simulink model "BLDC_Ctrl_MBD"  (R2020b)
settings: Solver=FixedStepDiscrete  StartTime=0.0  StopTime=10.0  FixedStep=0.0001  RelTol=1e-3
PreLoadFcn:
  | load('struct_BLDC_Crtl.mat');
InitFcn:
  | mbd_s32k_consistency_checks(bdroot(gcs));
undefined symbols (not defined in the file): External, LQFP, One, Shot, TRGMUX_PDB_TRIG
libraries: mbd_s32k1xx_ec_toolbox x34, mcbcontrolslib x4, mbd_msd_ec_toolbox x1
(part 1 of 2)
settings Model: Creator=k  LastModifiedBy=k
settings DataIOCC: ExternalInput=off  InitialState=off  SaveOutput=off  SignalLogging=off  SaveTime=off
settings OptimizationCC: DefaultParameterBehavior=Inlined  EnhancedBackFolding=on  PassReuseOutputArgsAs=Individual arguments  ZeroExternalMemoryAtStartup=off  ZeroInternalMemoryAtStartup=off  OptimizeBlockOrder=speed  DifferentSizesBufferReuse=on  OptimizationCustomize=off  EfficientTunableParamExpr=on
settings DebuggingCC: InheritedTsInSrcMsg=none  SingleTaskRateTransMsg=error  ParameterTunabilityLossMsg=error  UnconnectedInputMsg=error  UnconnectedOutputMsg=error  UnconnectedLineMsg=error  UnknownTsInhSupMsg=error
settings HardwareCC: ProdBitPerPointer=32  ProdBitPerSizeT=32  ProdBitPerPtrDiffT=32  ProdLargestAtomicInteger=Long  ProdLargestAtomicFloat=Double  ProdWordSize=32  ProdHWDeviceType=ARM Compatible->ARM Cortex
settings ModelReferenceCC: ModelReferenceNumInstancesAllowed=Single
settings SFSimCC: MATLABDynamicMemAlloc=off
settings RTWCC: Description=Model Based Design Toolbox S32K1xx Code Generation Target  SystemTargetFile=mbd_s32k.tlc  MakeCommand=mbd_s32k_make_rtw COPY_MDLREF_INCLUDES=0  TemplateMakefile=mbd_s32k.tmf  GenerateReport=on
settings CodeAppCC: ForceParamTrailComments=on  IgnoreCustomStorageClasses=off  OperatorAnnotations=on  SimulinkDataObjDesc=on  SFDataObjDesc=on  InsertBlockDesc=on
settings STFCustomTargetCC: TargetLangStandard=C99 (ISO)  MultiwordLength=256  ConcurrentExecutionCompliant=off  CombineOutputUpdateFcns=on  ERTCustomFileBanners=on  SupportContinuousTime=off  SupportNonInlinedSFcns=off  RemoveResetFunc=on  MATLABClassNameForMDSCustomization=Simulink.SoftwareTarget.ERTCustomization  CPPClassGenCompliant=off  GRTInterface=off  SystemTargetFile=mbd_s32k.tlc
settings ERTTargetCC: TargetLangStandard=C99 (ISO)  ParMdlRefBuildCompliant=off  CompOptLevelCompliant=off  ConcurrentExecutionCompliant=off  ModelStepFunctionPrototypeControlCompliant=off  CPPClassGenCompliant=off  UseToolchainInfoCompliant=off  InlinedParameterPlacement=NonHierarchical  ERTSrcFileBannerTemplate=mbd_ert_code_template.cgt  ERTHdrFileBannerTemplate=mbd_ert_code_template.cgt  ERTDataSrcFileTemplate=mbd_ert_code_template.cgt  ERTDataHdrFileTemplate=mbd_ert_code_template.cgt  ERTCustomFileTemplate=example_file_process.tlc

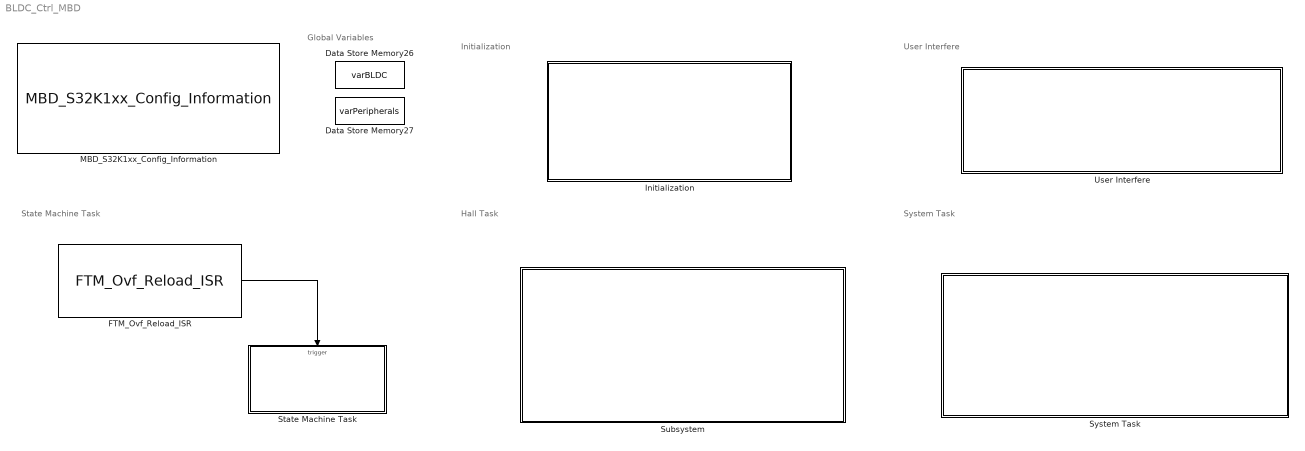
== system BLDC_Ctrl_MBD ==
  note: State Machine Task
  note: Global Variables
  note: Hall Task
  note: System Task
  note: Initialization
  note: User Interfere
  Data Store Memory26 : DataStoreMemory  DataStoreName=varBLDC  ReadBeforeWriteMsg=warning  WriteAfterWriteMsg=warning  WriteAfterReadMsg=warning  ShowAdditionalParam=off  OutDataTypeStr=Bus: structBLDC
  Data Store Memory27 : DataStoreMemory  DataStoreName=varPeripherals  ReadBeforeWriteMsg=warning  WriteAfterWriteMsg=warning  WriteAfterReadMsg=warning  ShowAdditionalParam=off  OutDataTypeStr=Bus: structPeripherals
  FTM_Ovf_Reload_ISR : mbd_s32k1xx_ec_toolbox/Motor Control Blocks/FTM Blocks/FTM_Ovf_Reload_ISR  Priority=10  ftmModule=3  mcuTargetUpdate=on
  Initialization : Subsystem
  MBD_S32K1xx_Config_Information : mbd_s32k1xx_ec_toolbox/MBD_S32K1xx_Config_Information  mbdt_ver=0  disp_str=|  config_params=[]  mcu_target_name=S32K144  mcu_target_package=100-LQFP  mcu_target_sram_size=64KB  mcu_system_clock_freq=80  mcu_xtal_freq=External 8  mcu_steptick_timer=LPIT Channel 0  mcu_steptick_prio=15  ds_import_enable=on  target_compiler=GCC  target_memory=FLASH  gcc_target_compile_opts=-mthumb -mfloat-abi=hard -mfpu=fpv4-sp-d16 -O1 -g -gstrict-dwarf  gcc_target_assemble_opts=-mthumb -mfloat-abi=hard -mfpu=fpv4-sp-d16 -g  gcc_target_link_opts=-mthumb -mfloat-abi=hard -mfpu=fpv4-sp-d16  gcc_target_default_lcf=on  gcc_target_user_lcf=S32K148_192_flash.ld  ghs_target_compile_opts=-cpu=cortexm4f -thumb -fpu=vfpv4_d16 -fsingle -Ogeneral -Wundef -Wimplicit-int -Wshadow -Wtrigraphs --no_commons --gnu_asm -gnu99 -gdwarf-2 -G  ghs_target_assemble_opts=-cpu=cortexm4f -fpu=vfpv4_d16  ghs_target_link_opts=-cpu=cortexm4f -thumb -fpu=vfpv4_d16  ghs_target_default_lcf=on  ghs_target_user_lcf=S32K148_192_flash.ld  iar_target_compile_opts=--cpu=Cortex-M4F --thumb --fpu=VFPv4_sp -Ol -e --debug --dlib_config normal  iar_target_assemble_opts=--cpu Cortex-M4F --thumb --fpu VFPv4_sp  iar_target_link_opts=--no_exceptions --vfe --inline  iar_target_default_lcf=on  iar_target_user_lcf=S32K148_192_flash.icf  pil_download_enable=off  rbl_download_enable=on  rbl_start_delay=5000  rbl_download_interface=OpenSDA  rbl_restart_request=off  rbl_com_port=Custom  rbl_com_port_custom=COM1  pil_download_rate=57600  pil_opensda_drive=Custom  pil_opensda_drive_custom=E  pil_uart_instance=1  pil_uart_rx=PTC6: [LPUART1_RX | Receive]  pil_uart_tx=PTC7: [LPUART1_TX | Transmit]  FTM_PWM_PcrCheckEnDis=on  FTM_Input_Edge_Inputs_PcrCheckEnDis=on  FTM_Dual_Edge_Inputs_PcrCheckEnDis=on  FTM_Quadrature_Inputs_PcrCheckEnDis=on  FTM_Hall_Sensor_Inputs_PcrCheckEnDis=on  LPTMR_PcrCheckEnDis=on  PIT_PcrCheckEnDis=on  RTC_PcrCheckEnDis=on  FlexCAN_PcrCheckEnDis=on  LIN_PcrCheckEnDis=on  FlexIO_PcrCheckEnDis=on  LPI2C_PcrCheckEnDis=on  LPSPI_PcrCheckEnDis=on  LPUART_PcrCheckEnDis=on  CMP_PcrCheckEnDis=on  GPIO_OutputPcrCheckEnDis=on  GPIO_InputPcrCheckEnDis=on  SBC_PcrCheckEnDis=on  BMS_PcrCheckEnDis=on  AMMCLIB_PcrCheckEnDis=on  FM_PcrCheckEnDis=on  Profile_PcrCheckEnDis=on  ConfigParams_PcrCheckEnDis=on  ModelRef_PcrCheckEnDis=on  PDB0_PcrCheckEnDis=on  CSEc_PcrCheckEnDis=on  eDMA_PcrCheckEnDis=on  FLASH_PcrCheckEnDis=on  ADC_PcrCheckEnDis=on  WDOG_PcrCheckEnDis=on
      | Target : S32K144-64KB_SRAM
      | Package : 100-pin
      | System clock : 80 MHz
      | XTAL clock : External 8 MHz
      | Compiler : IAR
      | Target Type : FLASH
      | Download Code after build : off
      | Step Tick Interrupt Priority : 15
  State Machine Task : Subsystem
  Subsystem : Subsystem
  System Task : Subsystem
  User Interfere : Subsystem
  wires:
  FTM_Ovf_Reload_ISR/1 -> State Machine Task/Trigger

== system BLDC_Ctrl_MBD/Initialization ==
  note: FreeMASTER
  note: ADC
  note: Configuration
  ADC_Config : mbd_s32k1xx_ec_toolbox/Motor Control Blocks/ADC Blocks/ADC_Config  instance=0  mode=12-bit conversion  smplts=20  adiclk=alternate clock 1  adiv=input clock  show_adv_opts=on  pretrgsel=PDB pre-trigger  swpretrg=Disabled  adtrg=hardware  trgsel=PDB output  refsel=Vrefh and Vrefl  supply_monitoring=off  acfe=off  acfgt=off  acren=off  cv1=0  cv2=0  adco=off  avge=off  avgs=4 samples
  ADC_Config1 : mbd_s32k1xx_ec_toolbox/Motor Control Blocks/ADC Blocks/ADC_Config  instance=1  mode=12-bit conversion  smplts=20  adiclk=alternate clock 1  adiv=input clock  show_adv_opts=on  pretrgsel=PDB pre-trigger  swpretrg=Disabled  adtrg=hardware  trgsel=PDB output  refsel=Vrefh and Vrefl  supply_monitoring=off  acfe=off  acfgt=off  acren=off  cv1=0  cv2=0  adco=off  avge=off  avgs=4 samples
  ADC_Interleave : mbd_s32k1xx_ec_toolbox/Motor Control Blocks/ADC Blocks/ADC_Interleave  adcInterleavePins=PTB1 to ADC0_SE5 and ADC1_SE15  adcInterleaveInit=on
  FreeMaster_Config : mbd_s32k1xx_ec_toolbox/Utility Blocks/FreeMaster_Config  interface=LPUART1  baudrate=115200  rxd=PTC6: [LPUART1_RX | Receive]  txd=PTC7: [LPUART1_TX | Transmit]  mode=Poll-driven  isr_prio=15  show_adv_opts=on  use_scope=on  max_scope_vars=8  use_recorder=on  max_rec_vars=8  rec_buff_size=8192  rec_timebase=50 milliseconds  comm_buffer_size_auto=on  comm_buffer_size=255  comm_rqueue_size_default=on  comm_rqueue_size=32
  "LPSPI_Config " : mbd_s32k1xx_ec_toolbox/Communication Blocks/SPI Blocks/LPSPI_Config   InstanceNumber=0  Role=Master  BaudRate=1000000  ShowAdvanced=on  sin=PTB3: [LPSPI0_SIN | LPSPI Serial Data Input]  sout=PTB4: [LPSPI0_SOUT | LPSPI Serial Data Output]  sck=PTB2: [LPSPI0_SCK | LPSPI Serial Clock I/O]  pcs0=None  pcs1=PTB5: [LPSPI0_PCS1 | Peripheral Chip Select 1]  pcs2=None  pcs3=None  CPHA=1  CPOL=0  BitOrder=MSB first  TransferSize=8  WhichPCS=0  PCSPol=ActiveLow  ContinuousTransfer=off
  PDB_Config : mbd_s32k1xx_ec_toolbox/Motor Control Blocks/PDB Blocks/PDB_Config  pdbModule=0  regScCont=One-Shot  regScTrgsel=External (TRGMUX_PDB_TRIG)  trgMuxSel=FTM3 Initialize Trigger  trgMuxSelPin=PTB5: [TRGMUX_IN0 | Trigger Mux Input]  regModModulus=3900  regScPrescaler=1  regScMult=1  regPoenPoen0=off  regPo0DlyDly1=0  regPo0DlyDly2=0  enable_pdb_init=on  show_adv_opts=on  regCh0C1En0=on  regCh0C1En1=on  regCh0C1En2=off  regCh0C1En3=off  regCh0C1En4=off  regCh0C1En5=off  regCh0C1En6=off  regCh0C1En7=off  regCh0C1Bb0=off  regCh0C1Bb1=off  regCh0C1Bb2=off  regCh0C1Bb3=off  regCh0C1Bb4=off  regCh0C1Bb5=off  regCh0C1Bb6=off  regCh0C1Bb7=off  regCh0C1Tos0=Pre-trigger is in delay mode  regCh0C1Tos1=Pre-trigger is in delay mode  regCh0C1Tos2=Pre-trigger is in delay mode  regCh0C1Tos3=Pre-trigger is in delay mode  regCh0C1Tos4=Pre-trigger is in delay mode  regCh0C1Tos5=Pre-trigger is in delay mode  regCh0C1Tos6=Pre-trigger is in delay mode  regCh0C1Tos7=Pre-trigger is in delay mode  regCh0DlyDly0=1500  regCh0DlyDly1=2000  regCh0DlyDly2=1000  regCh0DlyDly3=1500  regCh0DlyDly4=0  regCh0DlyDly5=0  regCh0DlyDly6=0  regCh0DlyDly7=0  regCh1C1En0=off  regCh1C1En1=off  regCh1C1En2=off  regCh1C1En3=off  regCh1C1En4=off  regCh1C1En5=off  regCh1C1En6=off  regCh1C1En7=off  regCh1C1Bb0=off  regCh1C1Bb1=off  regCh1C1Bb2=off  regCh1C1Bb3=off  regCh1C1Bb4=off  regCh1C1Bb5=off  regCh1C1Bb6=off  regCh1C1Bb7=off  regCh1C1Tos0=Pre-trigger is in delay mode  regCh1C1Tos1=Pre-trigger is in delay mode  regCh1C1Tos2=Pre-trigger is in delay mode  regCh1C1Tos3=Pre-trigger is in delay mode  regCh1C1Tos4=Pre-trigger is in delay mode  regCh1C1Tos5=Pre-trigger is in delay mode  regCh1C1Tos6=Pre-trigger is in delay mode  regCh1C1Tos7=Pre-trigger is in delay mode  regCh1DlyDly0=0  regCh1DlyDly1=0  regCh1DlyDly2=0  regCh1DlyDly3=0  regCh1DlyDly4=0  regCh1DlyDly5=0  regCh1DlyDly6=0  regCh1DlyDly7=0
  PDB_Config1 : mbd_s32k1xx_ec_toolbox/Motor Control Blocks/PDB Blocks/PDB_Config  pdbModule=1  regScCont=One-Shot  regScTrgsel=External (TRGMUX_PDB_TRIG)  trgMuxSel=FTM3 Initialize Trigger  trgMuxSelPin=PTB5: [TRGMUX_IN0 | Trigger Mux Input]  regModModulus=3900  regScPrescaler=1  regScMult=1  regPoenPoen0=off  regPo0DlyDly1=0  regPo0DlyDly2=0  enable_pdb_init=on  show_adv_opts=on  regCh0C1En0=on  regCh0C1En1=on  regCh0C1En2=on  regCh0C1En3=off  regCh0C1En4=off  regCh0C1En5=off  regCh0C1En6=off  regCh0C1En7=off  regCh0C1Bb0=off  regCh0C1Bb1=off  regCh0C1Bb2=off  regCh0C1Bb3=off  regCh0C1Bb4=off  regCh0C1Bb5=off  regCh0C1Bb6=off  regCh0C1Bb7=off  regCh0C1Tos0=Pre-trigger is in delay mode  regCh0C1Tos1=Pre-trigger is in delay mode  regCh0C1Tos2=Pre-trigger is in delay mode  regCh0C1Tos3=Pre-trigger is in delay mode  regCh0C1Tos4=Pre-trigger is in delay mode  regCh0C1Tos5=Pre-trigger is in delay mode  regCh0C1Tos6=Pre-trigger is in delay mode  regCh0C1Tos7=Pre-trigger is in delay mode  regCh0DlyDly0=1000  regCh0DlyDly1=1500  regCh0DlyDly2=2000  regCh0DlyDly3=0  regCh0DlyDly4=0  regCh0DlyDly5=0  regCh0DlyDly6=0  regCh0DlyDly7=0  regCh1C1En0=off  regCh1C1En1=off  regCh1C1En2=off  regCh1C1En3=off  regCh1C1En4=off  regCh1C1En5=off  regCh1C1En6=off  regCh1C1En7=off  regCh1C1Bb0=off  regCh1C1Bb1=off  regCh1C1Bb2=off  regCh1C1Bb3=off  regCh1C1Bb4=off  regCh1C1Bb5=off  regCh1C1Bb6=off  regCh1C1Bb7=off  regCh1C1Tos0=Pre-trigger is in delay mode  regCh1C1Tos1=Pre-trigger is in delay mode  regCh1C1Tos2=Pre-trigger is in delay mode  regCh1C1Tos3=Pre-trigger is in delay mode  regCh1C1Tos4=Pre-trigger is in delay mode  regCh1C1Tos5=Pre-trigger is in delay mode  regCh1C1Tos6=Pre-trigger is in delay mode  regCh1C1Tos7=Pre-trigger is in delay mode  regCh1DlyDly0=0  regCh1DlyDly1=0  regCh1DlyDly2=0  regCh1DlyDly3=0  regCh1DlyDly4=0  regCh1DlyDly5=0  regCh1DlyDly6=0  regCh1DlyDly7=0
  TPP_Config : mbd_msd_ec_toolbox/TPP/TPP_Config  Priority=1  tppInstance=0  desatMode=on  fullonMode=off  lockMode=off  overtempEvent=on  phaseEvent=off  desatEvent=off  framingEvent=on  vlsEvent=on  writeErrEvent=on  overcurrentEvent=on  resetEvent=on  mcuTppIntEn=off  prioInt=15  tppDeadtime=1500  initTppNow=on  tppSpiInst=Please add SPI block to workspace  tppPwmModule=Please add FTM block to workspace  tppPair0_1=on  tppPair2_3=on  tppPair4_5=on  tppPair6_7=off  tppFirstChHS=on  tppEn1Pin=PTA2: [PTA2 | Port A I/O]  tppEn2Pin=PTA2: [PTA2 | Port A I/O]  tppRstPin=PTA3: [PTA3 | Port A I/O]  tppCsPin=PTB5: [PTB5 | Port B I/O]  tppIntPin=PTE10: [PTE10 | Port E I/O]

== system BLDC_Ctrl_MBD/State Machine Task ==
  function : TriggerPort  TriggerType=function-call  VariantControl=Variant
  Chart : Stateflow chart  TreatAsAtomicUnit=on
      settings: PortSchema="{\"entries\":[{\"content\":{\"sides\":[{\"content\":{\"connectorIds\":[\"In1\",\"In2\"]},\"type\":\"ConnectorPlacement.EquallySpacedRectSide\",\"uuid\":\"6aab3670-dbd5-4778-9051-de706f320d6c\"},{\"content\":{\"connectorIds\":[\"Out7\",\"Out2\",\"Out3\",\"Out1\",\"Out4\",\"Out5\",\"Out6\",\"Out8\"],\"side\":\"RIGHT\"},\"type\":\"ConnectorPlacement.EquallySpacedRectSide\",\"uuid\":\"2f9f0170-7a01-4f36-b182-da63b20b6c86\"},{\"content\":{\"connectorIds\":[],\"side\":\"TOP\"},\"type\":\"ConnectorPlacement.EquallySpacedRectSide\",\"uuid\":\"ed2088fa-8282-455e-b501-bc381afe58e4\"},{\"content\":{\"connectorIds\":[],\"side\":\"HIDDEN\"},\"type\":\"ConnectorPlacement.EquallySpacedRectSide\",\"uuid\":\"d652818b-6052-4db5-9e3c-1b8d8b3f5bf8\"}]},\"type\":\"ConnectorPlacement.EquallySpacedConnector\",\"uuid\":\"e57e4f41-1290-4580-a9fc-0c62073a8c32\"}],\"packageUris\":[\"http://schema.mathworks.com/mf0/Connector/R2020b\"],\"version\":\"1.0\"}"
  Data Store Read1 : DataStoreRead  DataStoreName=varBLDC  DataStoreElements=varBLDC.varMotorCtrl.FaultSetClear
  Data Store Read3 : DataStoreRead  DataStoreName=varBLDC  DataStoreElements=varBLDC.varMotorCtrl.MotorOnOff
  FreeMaster_Recorder_Call : mbd_s32k1xx_ec_toolbox/Utility Blocks/FreeMaster_Recorder_Call
  Read ADC : Subsystem
  State Functions : Subsystem  Priority=1
  Update FTM : Subsystem
  wires:
  Chart/7(ReadADCFunc()) -> Read ADC/Trigger
  Data Store Read1/1 -> Chart/2(FaultSetClear)
  Chart/8(UpdateFTMFunc()) -> Update FTM/Trigger
  Chart/6(FaultFunc()) -> State Functions/6(FaultFuncCall)
  Chart/3(ReadyFunc()) -> State Functions/2(ReadyFuncCall)
  Chart/5(NormalRunFunc()) -> State Functions/5(NomalRunFuncCall)
  Chart/1(MeasFunc()) -> State Functions/3(MeasFuncCall)
  Chart/2(InitFunc()) -> State Functions/1(InitFuncCall)
  Chart/4(CalFunc()) -> State Functions/4(CalFuncCall)
  Data Store Read3/1 -> Chart/1(MotorOnOff)

== system BLDC_Ctrl_MBD/Subsystem ==
  Digital_Input_ISR : mbd_s32k1xx_ec_toolbox/GPIO Blocks/Digital_Input_ISR  gpio_pin=PTA1: [PTA1 | Port A I/O]  irqc=on either-edge  prio=5
  Digital_Input_ISR1 : mbd_s32k1xx_ec_toolbox/GPIO Blocks/Digital_Input_ISR  gpio_pin=PTA15: [PTA15 | Port A I/O]  irqc=on either-edge  prio=5
  Digital_Input_ISR2 : mbd_s32k1xx_ec_toolbox/GPIO Blocks/Digital_Input_ISR  gpio_pin=PTA16: [PTA16 | Port A I/O]  irqc=on either-edge  prio=5
  Hall A : Subsystem  TreatAsAtomicUnit=on
  Hall B : Subsystem  TreatAsAtomicUnit=on
  Hall C : Subsystem  TreatAsAtomicUnit=on
  wires:
  Digital_Input_ISR/1 -> Hall C/Trigger
  Digital_Input_ISR1/1 -> Hall A/Trigger
  Digital_Input_ISR2/1 -> Hall B/Trigger

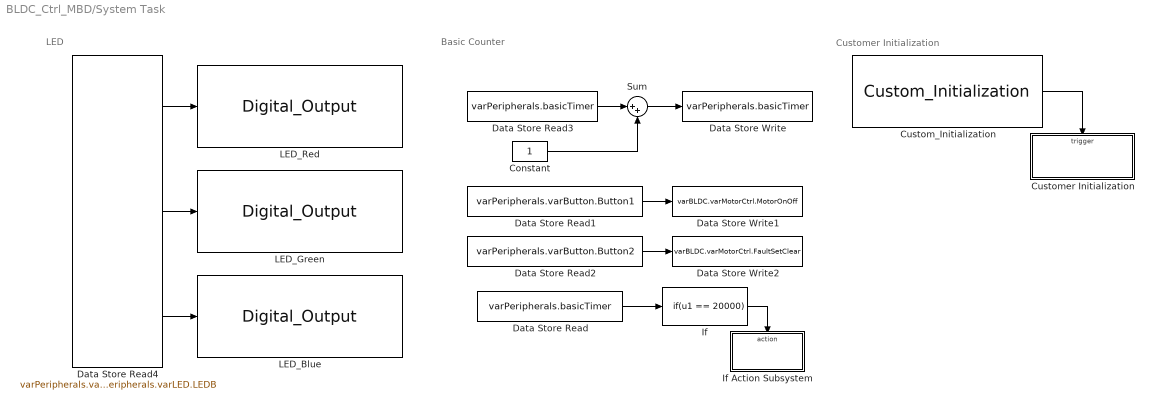
== system BLDC_Ctrl_MBD/System Task ==
  note: LED
  note: Basic Counter
  note: Customer Initialization
  Constant : Constant  OutDataTypeStr=uint32
  Custom_Initialization : mbd_s32k1xx_ec_toolbox/Utility Blocks/Custom_Initialization
  Customer Initialization : Subsystem  TreatAsAtomicUnit=on
  Data Store Read : DataStoreRead  DataStoreName=varPeripherals  DataStoreElements=varPeripherals.basicTimer
  Data Store Read1 : DataStoreRead  DataStoreName=varPeripherals  DataStoreElements=varPeripherals.varButton.Button1
  Data Store Read2 : DataStoreRead  DataStoreName=varPeripherals  DataStoreElements=varPeripherals.varButton.Button2
  Data Store Read3 : DataStoreRead  DataStoreName=varPeripherals  DataStoreElements=varPeripherals.basicTimer
  Data Store Read4 : DataStoreRead  DataStoreName=varPeripherals  DataStoreElements=varPeripherals.varLED.LEDR#varPeripherals.varLED.LEDG#varPeripherals.varLED.LEDB
  Data Store Write : DataStoreWrite  DataStoreName=varPeripherals  DataStoreElements=varPeripherals.basicTimer
  Data Store Write1 : DataStoreWrite  DataStoreName=varBLDC  DataStoreElements=varBLDC.varMotorCtrl.MotorOnOff
  Data Store Write2 : DataStoreWrite  DataStoreName=varBLDC  DataStoreElements=varBLDC.varMotorCtrl.FaultSetClear
  If : If  IfExpression=u1 == 20000  ShowElse=off
  If Action Subsystem : Subsystem  TreatAsAtomicUnit=on
  LED_Blue : mbd_s32k1xx_ec_toolbox/GPIO Blocks/Digital_Output  gpio_pin=PTD0: [PTD0 | Port D I/O]  init_val=High  drive_strength=Low
  LED_Green : mbd_s32k1xx_ec_toolbox/GPIO Blocks/Digital_Output  gpio_pin=PTD16: [PTD16 | Port D I/O]  init_val=High  drive_strength=Low
  LED_Red : mbd_s32k1xx_ec_toolbox/GPIO Blocks/Digital_Output  gpio_pin=PTD15: [PTD15 | Port D I/O]  init_val=High  drive_strength=Low
  Sum : Sum  Inputs=|++
  wires:
  Data Store Read4/1 -> LED_Red/1
  Data Store Read4/2 -> LED_Green/1
  Data Store Read4/3 -> LED_Blue/1
  Constant/1 -> Sum/2
  Sum/1 -> Data Store Write/1
  Custom_Initialization/1 -> Customer Initialization/Trigger
  Data Store Read1/1 -> Data Store Write1/1
  Data Store Read2/1 -> Data Store Write2/1
  Data Store Read/1 -> If/1
  If/1 -> If Action Subsystem/Action
  Data Store Read3/1 -> Sum/1

== system BLDC_Ctrl_MBD/User Interfere ==
  note: User Button
  note: User PIT Task
  Digital_Input_ISR : mbd_s32k1xx_ec_toolbox/GPIO Blocks/Digital_Input_ISR  gpio_pin=PTC12: [PTC12 | Port C I/O]  irqc=on rising-edge  prio=13
  Digital_Input_ISR1 : mbd_s32k1xx_ec_toolbox/GPIO Blocks/Digital_Input_ISR  gpio_pin=PTC13: [PTC13 | Port C I/O]  irqc=on rising-edge  prio=13
  Function-Call Subsystem1 : Subsystem  TreatAsAtomicUnit=on
  Function-Call Subsystem2 : Subsystem  TreatAsAtomicUnit=on
  Periodic_Interrupt_Timer : mbd_s32k1xx_ec_toolbox/Utility Blocks/Periodic_Interrupt_Timer  channel=1  period=200  prio=14  startCounter=on
  User PIT Task : Subsystem  TreatAsAtomicUnit=on
  wires:
  Digital_Input_ISR/1 -> Function-Call Subsystem2/Trigger
  Digital_Input_ISR1/1 -> Function-Call Subsystem1/Trigger
  Periodic_Interrupt_Timer/1 -> User PIT Task/Trigger

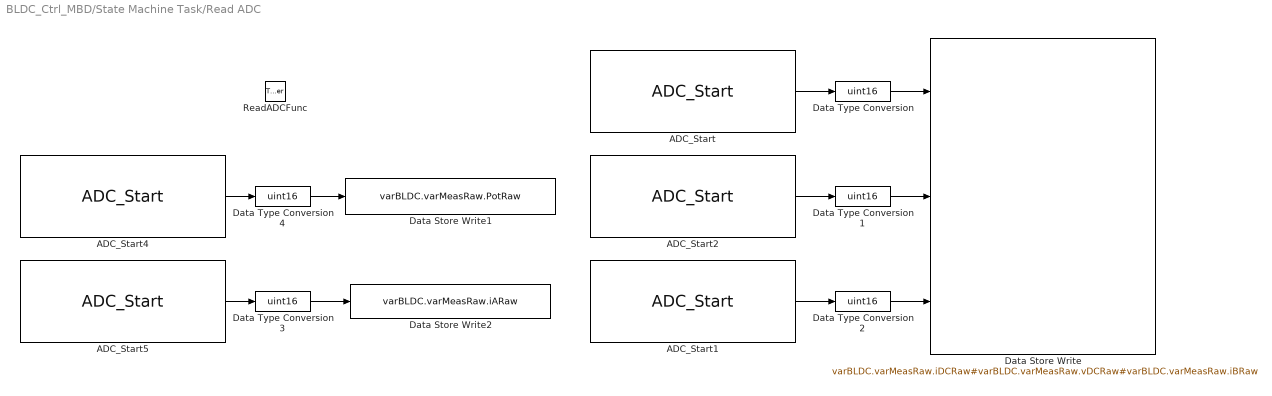
== system BLDC_Ctrl_MBD/State Machine Task/Read ADC ==
  ReadADCFunc : TriggerPort  TriggerType=function-call  VariantControl=Variant
  ADC_Start : mbd_s32k1xx_ec_toolbox/Motor Control Blocks/ADC Blocks/ADC_Start  instance=1  adc_r=A  adc_chan=PTD4: [ADC1_SE6 | ADC Single Ended Input]  aien=off  mcuTargetUpdate=on
  ADC_Start1 : mbd_s32k1xx_ec_toolbox/Motor Control Blocks/ADC Blocks/ADC_Start  instance=1  adc_r=C  adc_chan=PTB1: [ADC1_SE15 | ADC Single Ended Input]  aien=off  mcuTargetUpdate=on
  ADC_Start2 : mbd_s32k1xx_ec_toolbox/Motor Control Blocks/ADC Blocks/ADC_Start  instance=1  adc_r=B  adc_chan=PTB12: [ADC1_SE7 | ADC Single Ended Input]  aien=off  mcuTargetUpdate=on
  ADC_Start4 : mbd_s32k1xx_ec_toolbox/Motor Control Blocks/ADC Blocks/ADC_Start  instance=0  adc_r=A  adc_chan=PTC14: [ADC0_SE12 | ADC Single Ended Input]  aien=off  mcuTargetUpdate=on
  ADC_Start5 : mbd_s32k1xx_ec_toolbox/Motor Control Blocks/ADC Blocks/ADC_Start  instance=0  adc_r=B  adc_chan=PTB0: [ADC0_SE4 | ADC Single Ended Input]  aien=off  mcuTargetUpdate=on
  Data Store Write : DataStoreWrite  DataStoreName=varBLDC  DataStoreElements=varBLDC.varMeasRaw.iDCRaw#varBLDC.varMeasRaw.vDCRaw#varBLDC.varMeasRaw.iBRaw
  Data Store Write1 : DataStoreWrite  DataStoreName=varBLDC  DataStoreElements=varBLDC.varMeasRaw.PotRaw
  Data Store Write2 : DataStoreWrite  DataStoreName=varBLDC  DataStoreElements=varBLDC.varMeasRaw.iARaw
  Data Type Conversion{,1..4} (5 alike) : DataTypeConversion  OutDataTypeStr=uint16
  wires:
  ADC_Start5/1 -> Data Type Conversion3/1
  ADC_Start/1 -> Data Type Conversion/1
  ADC_Start1/1 -> Data Type Conversion2/1
  Data Type Conversion/1 -> Data Store Write/1
  ADC_Start4/1 -> Data Type Conversion4/1
  Data Type Conversion4/1 -> Data Store Write1/1
  ADC_Start2/1 -> Data Type Conversion1/1
  Data Type Conversion3/1 -> Data Store Write2/1
  Data Type Conversion2/1 -> Data Store Write/3
  Data Type Conversion1/1 -> Data Store Write/2

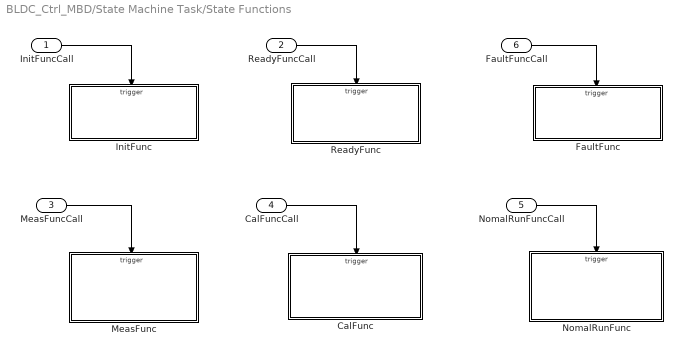
== system BLDC_Ctrl_MBD/State Machine Task/State Functions ==
  InitFuncCall : Inport
  ReadyFuncCall : Inport  Port=2
  MeasFuncCall : Inport  Port=3
  CalFuncCall : Inport  Port=4
  NomalRunFuncCall : Inport  Port=5
  FaultFuncCall : Inport  Port=6
  CalFunc : Subsystem  TreatAsAtomicUnit=on
  FaultFunc : Subsystem  TreatAsAtomicUnit=on
  InitFunc : Subsystem  TreatAsAtomicUnit=on
  MeasFunc : Subsystem  TreatAsAtomicUnit=on
  NomalRunFunc : Subsystem  TreatAsAtomicUnit=on
  ReadyFunc : Subsystem  TreatAsAtomicUnit=on
  wires:
  MeasFuncCall/1 -> MeasFunc/Trigger
  CalFuncCall/1 -> CalFunc/Trigger
  InitFuncCall/1 -> InitFunc/Trigger
  ReadyFuncCall/1 -> ReadyFunc/Trigger
  FaultFuncCall/1 -> FaultFunc/Trigger
  NomalRunFuncCall/1 -> NomalRunFunc/Trigger

== system BLDC_Ctrl_MBD/State Machine Task/Update FTM ==
  UpdateFTMFunc : TriggerPort  TriggerType=function-call  VariantControl=Variant
  Data Store Read2 : DataStoreRead  DataStoreName=varBLDC  DataStoreElements=varBLDC.varDuty.DutyA#varBLDC.varDuty.DutyB#varBLDC.varDuty.DutyC#varBLDC.varDuty.SWOCTRLcode#varBLDC.varDuty.OUTMASKcode
  FTM_PWM_Config : mbd_s32k1xx_ec_toolbox/Motor Control Blocks/FTM Blocks/FTM_PWM_Config  Priority=5  ftmModule=3  ftmMode=Center-Aligned PWM  ftmSourceClock=80 MHz  swcontrol_enable=on  chan0En=on  chan0Type=Complementary  chan2En=on  chan2Type=Complementary  chan4En=on  chan4Type=Complementary  chan6En=off  chan6Type=Independent  ftmPwmUnits=Hz  outFrequency=20000  ftmPeriod=4000  ftmPrescaler=Divide by 1  deadtimeUnits=Nanoseconds  deadtimeNs=1200  deadtimeTicks=24  deadtimePrescaler=Divide by 4  dutyCycleCh0=0  dutyCycleCh1=0  dutyCycleCh2=0  dutyCycleCh3=0  dutyCycleCh4=0  dutyCycleCh5=0  dutyCycleCh6=0.25  dutyCycleCh7=0.25  dutyCycleSim=off  startAfterInit=off  showAdvOpt=on  pinFtmCh0=PTB8: [FTM3_CH0 | FTM Channel]  pinFtmCh1=PTB9: [FTM3_CH1 | FTM Channel]  pinPolCh0=Active Low  pinPolCh1=Active Low  outputComplem0=Main duplicated  outputLevel0=High  outputLevel1=Low  pinFtmCh2=PTB10: [FTM3_CH2 | FTM Channel]  pinFtmCh3=PTB11: [FTM3_CH3 | FTM Channel]  pinPolCh2=Active Low  pinPolCh3=Active Low  outputComplem2=Main duplicated  outputLevel2=High  outputLevel3=Low  pinFtmCh4=PTC10: [FTM3_CH4 | FTM Channel]  pinFtmCh5=PTC11: [FTM3_CH5 | FTM Channel]  pinPolCh4=Active Low  pinPolCh5=Active Low  outputComplem4=Main duplicated  outputLevel4=High  outputLevel5=Low  pinFtmCh6=PTC12: [FTM3_CH6 | FTM Channel]  pinFtmCh7=None  pinPolCh6=Active Low  pinPolCh7=Active Low  outputComplem6=Main duplicated  outputLevel6=Low  outputLevel7=Low  initTrigger=off  chTrigger0=off  chTrigger1=off  chTrigger2=off  chTrigger3=off  chTrigger4=off  chTrigger5=off  chTrigger6=off  chTrigger7=off  mcuTargetUpdate=on  pwmSyncTrg=Software trigger  pwmSyncHwRouting=TRGMUX_FTM7  pwmSyncTrg0=off  pwmSyncTrg1=off  pwmSyncTrg2=off  pwmSyncAutoClear=off  pwmSyncMinLoad=on  pwmSyncMaxLoad=off  pwmSyncInvert=PWM Syncronization  pwmSyncOutControl=System Clock  pwmSyncOutMask=System Clock  pwmSyncCounterInitial=PWM Syncronization  pwmSyncPoints=Wait Loading Points  reloadEnable=on  reloadPriority=5  reloadHalfCycle=off  reloadHCR=0  reloadFrequency=0  chnMatch0=off  chnMatch1=off  chnMatch2=off  chnMatch3=off  chnMatch4=off  chnMatch5=off  chnMatch6=off  chnMatch7=off  pwmFaultProtection=off  pwmFaultInterrupt=off  pwmFaultClearing=Fault control disabled  pwmFaultPinState=Safe Value  pwmFaultFilterValue=0  pwmFaultPriority=15  fault_disen_0=off  fault_filter_0=off  fault_polarity_0=Active High  fault_disen_1=off  fault_filter_1=off  fault_polarity_1=Active high  fault_disen_2=off  fault_filter_2=off  fault_polarity_2=Active high  fault_disen_3=off  fault_filter_3=off  fault_polarity_3=Active high  fault_pin_0=None  fault_pin_1=None  fault_pin_2=None  fault_pin_3=None
  wires:
  Data Store Read2/1 -> FTM_PWM_Config/1
  Data Store Read2/3 -> FTM_PWM_Config/3
  Data Store Read2/2 -> FTM_PWM_Config/2
  Data Store Read2/4 -> FTM_PWM_Config/4
  Data Store Read2/5 -> FTM_PWM_Config/5

== system BLDC_Ctrl_MBD/Subsystem/Hall A ==
  ReadHallA : TriggerPort  TriggerType=function-call  VariantControl=Variant
  Data Store Read1 : DataStoreRead  DataStoreName=varBLDC  DataStoreElements=varBLDC.varHallCalc.HallEnd
  Data Store Read5 : DataStoreRead  DataStoreName=varPeripherals  DataStoreElements=varPeripherals.basicTimer
  Data Store Write1 : DataStoreWrite  DataStoreName=varBLDC  DataStoreElements=varBLDC.varHall.HallA
  Data Store Write2 : DataStoreWrite  DataStoreName=varBLDC  DataStoreElements=varBLDC.varHallCalc.HallEnd
  Data Store Write3 : DataStoreWrite  DataStoreName=varBLDC  DataStoreElements=varBLDC.varHallCalc.HallStart
  Digital_Input_HALL_A : mbd_s32k1xx_ec_toolbox/GPIO Blocks/Digital_Input  gpio_pin=PTA15: [PTA15 | Port A I/O]  pull_resistor=None  passive_filter=off
  wires:
  Digital_Input_HALL_A/1 -> Data Store Write1/1
  Data Store Read1/1 -> Data Store Write3/1
  Data Store Read5/1 -> Data Store Write2/1

== system BLDC_Ctrl_MBD/Subsystem/Hall B ==
  ReadHallA : TriggerPort  TriggerType=function-call  VariantControl=Variant
  Data Store Read1 : DataStoreRead  DataStoreName=varBLDC  DataStoreElements=varBLDC.varHallCalc.HallEnd
  Data Store Read5 : DataStoreRead  DataStoreName=varPeripherals  DataStoreElements=varPeripherals.basicTimer
  Data Store Write1 : DataStoreWrite  DataStoreName=varBLDC  DataStoreElements=varBLDC.varHall.HallB
  Data Store Write2 : DataStoreWrite  DataStoreName=varBLDC  DataStoreElements=varBLDC.varHallCalc.HallEnd
  Data Store Write3 : DataStoreWrite  DataStoreName=varBLDC  DataStoreElements=varBLDC.varHallCalc.HallStart
  Digital_Input_HALL_B : mbd_s32k1xx_ec_toolbox/GPIO Blocks/Digital_Input  gpio_pin=PTA16: [PTA16 | Port A I/O]  pull_resistor=None  passive_filter=off
  wires:
  Digital_Input_HALL_B/1 -> Data Store Write1/1
  Data Store Read5/1 -> Data Store Write2/1
  Data Store Read1/1 -> Data Store Write3/1

== system BLDC_Ctrl_MBD/Subsystem/Hall C ==
  ReadHallA : TriggerPort  TriggerType=function-call  VariantControl=Variant
  Data Store Read1 : DataStoreRead  DataStoreName=varBLDC  DataStoreElements=varBLDC.varHallCalc.HallEnd
  Data Store Read5 : DataStoreRead  DataStoreName=varPeripherals  DataStoreElements=varPeripherals.basicTimer
  Data Store Write1 : DataStoreWrite  DataStoreName=varBLDC  DataStoreElements=varBLDC.varHall.HallC
  Data Store Write2 : DataStoreWrite  DataStoreName=varBLDC  DataStoreElements=varBLDC.varHallCalc.HallEnd
  Data Store Write3 : DataStoreWrite  DataStoreName=varBLDC  DataStoreElements=varBLDC.varHallCalc.HallStart
  Digital_Input_HALL_C : mbd_s32k1xx_ec_toolbox/GPIO Blocks/Digital_Input  gpio_pin=PTA1: [PTA1 | Port A I/O]  pull_resistor=None  passive_filter=off
  wires:
  Digital_Input_HALL_C/1 -> Data Store Write1/1
  Data Store Read5/1 -> Data Store Write2/1
  Data Store Read1/1 -> Data Store Write3/1

== system BLDC_Ctrl_MBD/System Task/Customer Initialization ==
  CustInit : TriggerPort  TriggerType=function-call  VariantControl=Variant
  0_uint32 : Constant  Value=0  OutDataTypeStr=uint32
  1_boolean : Constant  OutDataTypeStr=boolean
  Data Store Write : DataStoreWrite  DataStoreName=varPeripherals  DataStoreElements=varPeripherals.varLED.LEDR#varPeripherals.varLED.LEDG#varPeripherals.varLED.LEDB#varPeripherals.basicTimer
  wires:
  1_boolean/1 -> Data Store Write/1, Data Store Write/2, Data Store Write/3
  0_uint32/1 -> Data Store Write/4

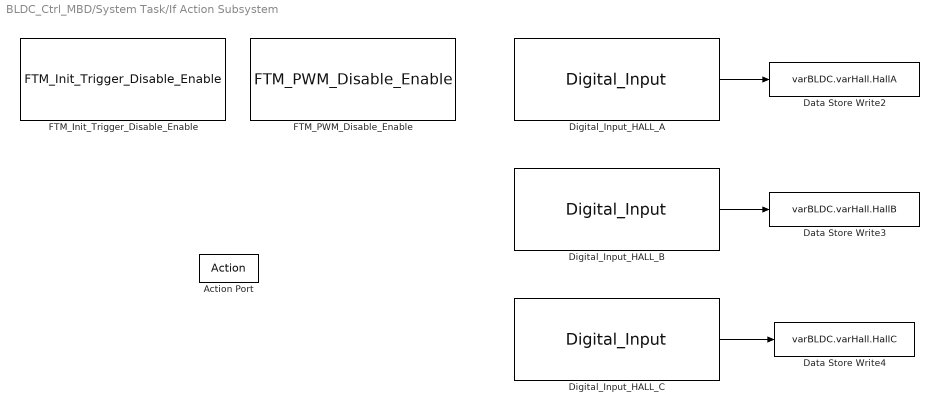
== system BLDC_Ctrl_MBD/System Task/If Action Subsystem ==
  Action Port : ActionPort  ActionPortLabel=if(u1 == 20000)
  Data Store Write2 : DataStoreWrite  DataStoreName=varBLDC  DataStoreElements=varBLDC.varHall.HallA
  Data Store Write3 : DataStoreWrite  DataStoreName=varBLDC  DataStoreElements=varBLDC.varHall.HallB
  Data Store Write4 : DataStoreWrite  DataStoreName=varBLDC  DataStoreElements=varBLDC.varHall.HallC
  Digital_Input_HALL_A : mbd_s32k1xx_ec_toolbox/GPIO Blocks/Digital_Input  gpio_pin=PTA15: [PTA15 | Port A I/O]  pull_resistor=None  passive_filter=off
  Digital_Input_HALL_B : mbd_s32k1xx_ec_toolbox/GPIO Blocks/Digital_Input  gpio_pin=PTA16: [PTA16 | Port A I/O]  pull_resistor=None  passive_filter=off
  Digital_Input_HALL_C : mbd_s32k1xx_ec_toolbox/GPIO Blocks/Digital_Input  gpio_pin=PTA1: [PTA1 | Port A I/O]  pull_resistor=None  passive_filter=off
  FTM_Init_Trigger_Disable_Enable : mbd_s32k1xx_ec_toolbox/Motor Control Blocks/FTM Blocks/FTM_Init_Trigger_Disable_Enable  ftmModule=3  action=Enable
  FTM_PWM_Disable_Enable : mbd_s32k1xx_ec_toolbox/Motor Control Blocks/FTM Blocks/FTM_PWM_Disable_Enable  ftmModule=3  action=Enable
  wires:
  Digital_Input_HALL_A/1 -> Data Store Write2/1
  Digital_Input_HALL_B/1 -> Data Store Write3/1
  Digital_Input_HALL_C/1 -> Data Store Write4/1

== system BLDC_Ctrl_MBD/User Interfere/Function-Call Subsystem1 ==
  function : TriggerPort  TriggerType=function-call  VariantControl=Variant
  Data Store Read : DataStoreRead  DataStoreName=varPeripherals  DataStoreElements=varPeripherals.varButton.Button2
  Data Store Write : DataStoreWrite  DataStoreName=varPeripherals  DataStoreElements=varPeripherals.varButton.Button2
  Logical Operator : Logic  Operator=NOT  AllPortsSameDT=off  OutDataTypeStr=boolean
  wires:
  Data Store Read/1 -> Logical Operator/1
  Logical Operator/1 -> Data Store Write/1

== system BLDC_Ctrl_MBD/User Interfere/Function-Call Subsystem2 ==
  function : TriggerPort  TriggerType=function-call  VariantControl=Variant
  Data Store Read : DataStoreRead  DataStoreName=varPeripherals  DataStoreElements=varPeripherals.varButton.Button1
  Data Store Write : DataStoreWrite  DataStoreName=varPeripherals  DataStoreElements=varPeripherals.varButton.Button1
  Logical Operator : Logic  Operator=NOT  AllPortsSameDT=off  OutDataTypeStr=boolean
  wires:
  Logical Operator/1 -> Data Store Write/1
  Data Store Read/1 -> Logical Operator/1

== system BLDC_Ctrl_MBD/User Interfere/User PIT Task ==
  UserPITFunc : TriggerPort  TriggerType=function-call  VariantControl=Variant
  Constant : Constant  Value=0.168  OutDataTypeStr=single
  Data Store Read : DataStoreRead  DataStoreName=varBLDC  DataStoreElements=varBLDC.varMeasRaw.PotRaw
  Data Store Write1 : DataStoreWrite  DataStoreName=varBLDC  DataStoreElements=varBLDC.varMotorCtrl.SpdReq
  Data Type Conversion : DataTypeConversion  OutDataTypeStr=single
  Product : Product
  Saturation : Saturate  UpperLimit=650  LowerLimit=0
  wires:
  Saturation/1 -> Data Store Write1/1
  Data Store Read/1 -> Data Type Conversion/1
  Data Type Conversion/1 -> Product/1
  Constant/1 -> Product/2
  Product/1 -> Saturation/1

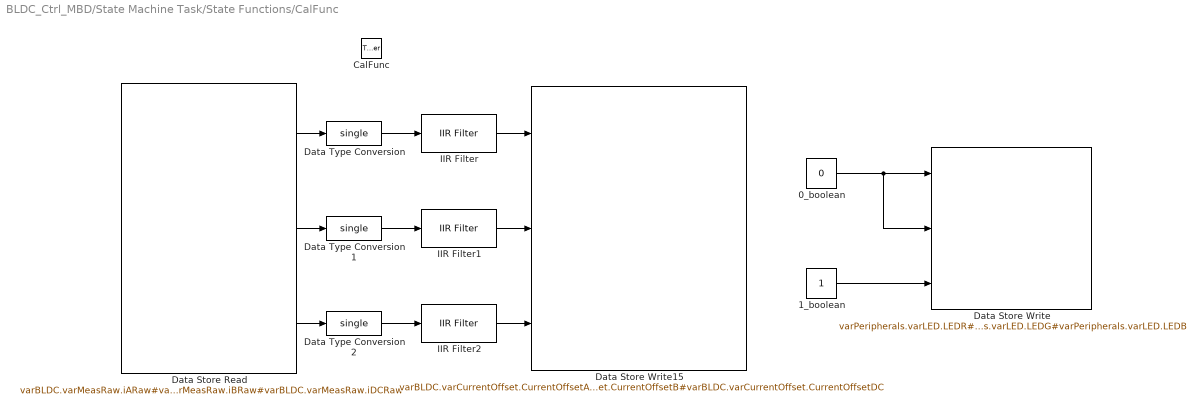
== system BLDC_Ctrl_MBD/State Machine Task/State Functions/CalFunc ==
  CalFunc : TriggerPort  TriggerType=function-call  VariantControl=Variant
  0_boolean : Constant  Value=0  OutDataTypeStr=boolean
  1_boolean : Constant  OutDataTypeStr=boolean
  Data Store Read : DataStoreRead  DataStoreName=varBLDC  DataStoreElements=varBLDC.varMeasRaw.iARaw#varBLDC.varMeasRaw.iBRaw#varBLDC.varMeasRaw.iDCRaw
  Data Store Write : DataStoreWrite  DataStoreName=varPeripherals  DataStoreElements=varPeripherals.varLED.LEDR#varPeripherals.varLED.LEDG#varPeripherals.varLED.LEDB
  Data Store Write15 : DataStoreWrite  DataStoreName=varBLDC  DataStoreElements=varBLDC.varCurrentOffset.CurrentOffsetA#varBLDC.varCurrentOffset.CurrentOffsetB#varBLDC.varCurrentOffset.CurrentOffsetDC
  Data Type Conversion : DataTypeConversion  OutDataTypeStr=single
  Data Type Conversion1 : DataTypeConversion  OutDataTypeStr=single
  Data Type Conversion2 : DataTypeConversion  OutDataTypeStr=single
  IIR Filter : mcbcontrolslib/IIR Filter  Filter_constant=0.001
      settings: SourceProductBaseCode=MT
  IIR Filter1 : mcbcontrolslib/IIR Filter  Filter_constant=0.001
      settings: SourceProductBaseCode=MT
  IIR Filter2 : mcbcontrolslib/IIR Filter  Filter_constant=0.001
      settings: SourceProductBaseCode=MT
  wires:
  Data Store Read/1 -> Data Type Conversion/1
  Data Store Read/2 -> Data Type Conversion1/1
  Data Store Read/3 -> Data Type Conversion2/1
  1_boolean/1 -> Data Store Write/3
  0_boolean/1 -> Data Store Write/2, Data Store Write/1
  IIR Filter/1 -> Data Store Write15/1
  IIR Filter1/1 -> Data Store Write15/2
  IIR Filter2/1 -> Data Store Write15/3
  Data Type Conversion/1 -> IIR Filter/1
  Data Type Conversion1/1 -> IIR Filter1/1
  Data Type Conversion2/1 -> IIR Filter2/1

== system BLDC_Ctrl_MBD/State Machine Task/State Functions/FaultFunc ==
  FaultFunc : TriggerPort  TriggerType=function-call  VariantControl=Variant
  Data Store Write : DataStoreWrite  DataStoreName=varPeripherals  DataStoreElements=varPeripherals.varLED.LEDR#varPeripherals.varLED.LEDG#varPeripherals.varLED.LEDB
  Data Store Write1 : DataStoreWrite  DataStoreName=varBLDC  DataStoreElements=varBLDC.varDuty.DutyA#varBLDC.varDuty.DutyB#varBLDC.varDuty.DutyC
  boolean0 : Constant  Value=0  OutDataTypeStr=boolean
  boolean1 : Constant  OutDataTypeStr=boolean
  single : Constant  Value=0  OutDataTypeStr=single
  wires:
  single/1 -> Data Store Write1/1, Data Store Write1/2, Data Store Write1/3
  boolean1/1 -> Data Store Write/3, Data Store Write/2
  boolean0/1 -> Data Store Write/1

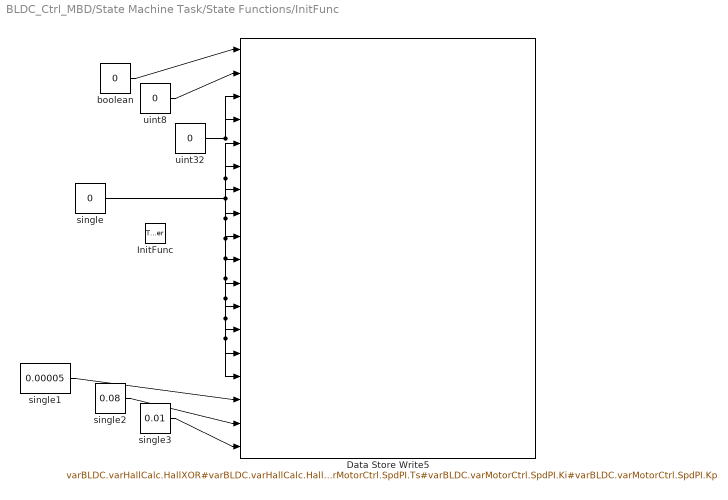
== system BLDC_Ctrl_MBD/State Machine Task/State Functions/InitFunc ==
  InitFunc : TriggerPort  TriggerType=function-call  VariantControl=Variant
  Data Store Write5 : DataStoreWrite  DataStoreName=varBLDC  DataStoreElements=varBLDC.varHallCalc.HallXOR#varBLDC.varHallCalc.HallSum#varBLDC.varHallCalc.HallStart#varBLDC.varHallCalc.HallEnd#varBLDC.varHallCalc.HallSpd#varBLDC.varCurrent.CurrentA#varBLDC.varCurrent.CurrentB#varBLDC.varCurrent.CurrentC#varBLDC.varCurrent.CurrentDC#varBLDC.varCurrentOffset.CurrentOffsetA#varBLDC.varCurrentOffset.CurrentOffsetB#varBLDC.varCurrentOffset.CurrentOffsetDC#varBLDC.varDuty.DutyA#varBLDC.varDuty.DutyB#varBLDC.varDuty.DutyC#varBLDC.varMotorCtrl.SpdPI.Ts#varBLDC.varMotorCtrl.SpdPI.Ki#varBLDC.varMotorCtrl.SpdPI.Kp
  boolean : Constant  Value=0  OutDataTypeStr=boolean
  single : Constant  Value=0  OutDataTypeStr=single
  single1 : Constant  Value=0.00005  OutDataTypeStr=single
  single2 : Constant  Value=0.08  OutDataTypeStr=single
  single3 : Constant  Value=0.01  OutDataTypeStr=single
  uint32 : Constant  Value=0  OutDataTypeStr=uint32
  uint8 : Constant  Value=0  OutDataTypeStr=uint8
  wires:
  boolean/1 -> Data Store Write5/1
  uint8/1 -> Data Store Write5/2
  single/1 -> Data Store Write5/5, Data Store Write5/6, Data Store Write5/15, Data Store Write5/14, Data Store Write5/13, Data Store Write5/12, Data Store Write5/11, Data Store Write5/10, Data Store Write5/9, Data Store Write5/8, Data Store Write5/7
  uint32/1 -> Data Store Write5/3, Data Store Write5/4
  single3/1 -> Data Store Write5/18
  single2/1 -> Data Store Write5/17
  single1/1 -> Data Store Write5/16

== system BLDC_Ctrl_MBD/State Machine Task/State Functions/MeasFunc ==
  MeasFunc : TriggerPort  TriggerType=function-call  VariantControl=Variant
  Current Calc : Subsystem  Priority=1
  Hall Calc : Subsystem  Priority=2
  Speed Calc : Subsystem

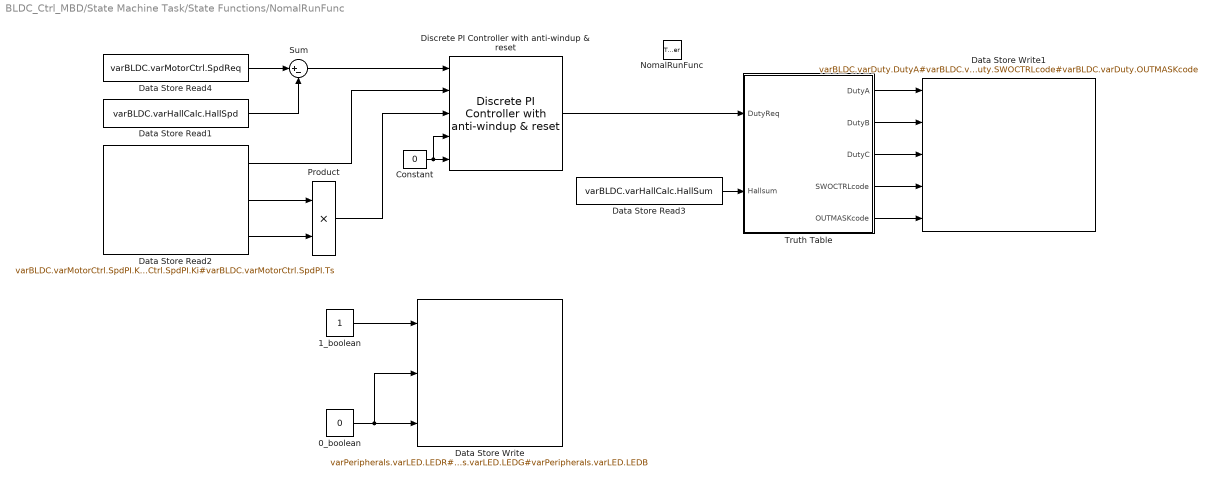
== system BLDC_Ctrl_MBD/State Machine Task/State Functions/NomalRunFunc ==
  NomalRunFunc : TriggerPort  TriggerType=function-call  VariantControl=Variant
  0_boolean : Constant  Value=0  OutDataTypeStr=boolean
  1_boolean : Constant  OutDataTypeStr=boolean
  Constant : Constant  Value=0  OutDataTypeStr=single
  Data Store Read1 : DataStoreRead  DataStoreName=varBLDC  DataStoreElements=varBLDC.varHallCalc.HallSpd
  Data Store Read2 : DataStoreRead  DataStoreName=varBLDC  DataStoreElements=varBLDC.varMotorCtrl.SpdPI.Kp#varBLDC.varMotorCtrl.SpdPI.Ki#varBLDC.varMotorCtrl.SpdPI.Ts
  Data Store Read3 : DataStoreRead  DataStoreName=varBLDC  DataStoreElements=varBLDC.varHallCalc.HallSum
  Data Store Read4 : DataStoreRead  DataStoreName=varBLDC  DataStoreElements=varBLDC.varMotorCtrl.SpdReq
  Data Store Write : DataStoreWrite  DataStoreName=varPeripherals  DataStoreElements=varPeripherals.varLED.LEDR#varPeripherals.varLED.LEDG#varPeripherals.varLED.LEDB
  Data Store Write1 : DataStoreWrite  DataStoreName=varBLDC  DataStoreElements=varBLDC.varDuty.DutyA#varBLDC.varDuty.DutyB#varBLDC.varDuty.DutyC#varBLDC.varDuty.SWOCTRLcode#varBLDC.varDuty.OUTMASKcode
  Discrete PI Controller with anti-windup & reset : mcbcontrolslib/Discrete PI Controller  with anti-windup & reset  UpperSaturationLimit=0.9  LowerSaturationLimit=0.1
      settings: SourceProductBaseCode=MT
  Product : Product
  Sum : Sum  Inputs=|+-
  Truth Table : Truth Table  TreatAsAtomicUnit=on
      settings: PortSchema="{\"entries\":[{\"content\":{\"sides\":[{\"content\":{\"connectorIds\":[\"In2\",\"In1\"]},\"type\":\"ConnectorPlacement.EquallySpacedRectSide\",\"uuid\":\"59c0d94d-4ab6-4082-9c20-9efdae7878b3\"},{\"content\":{\"connectorIds\":[\"Out1\",\"Out2\",\"Out3\",\"Out4\",\"Out5\"],\"side\":\"RIGHT\"},\"type\":\"ConnectorPlacement.EquallySpacedRectSide\",\"uuid\":\"fbebaf7f-5920-4df9-84a7-9b0467c91c72\"},{\"content\":{\"connectorIds\":[],\"side\":\"TOP\"},\"type\":\"ConnectorPlacement.EquallySpacedRectSide\",\"uuid\":\"8ff1c87b-d4dc-46a0-9459-25a6278b9f20\"},{\"content\":{\"connectorIds\":[],\"side\":\"HIDDEN\"},\"type\":\"ConnectorPlacement.EquallySpacedRectSide\",\"uuid\":\"16bdd2e1-f1a8-43ed-aa1c-d33053eb9e05\"}]},\"type\":\"ConnectorPlacement.EquallySpacedConnector\",\"uuid\":\"7896656f-e18e-44d5-80e3-9050e65d4579\"}],\"packageUris\":[\"http://schema.mathworks.com/mf0/Connector/R2020b\"],\"version\":\"1.0\"}"
  wires:
  Data Store Read3/1 -> Truth Table/1(Hallsum)
  Truth Table/1(DutyA) -> Data Store Write1/1
  Truth Table/2(DutyB) -> Data Store Write1/2
  Truth Table/3(DutyC) -> Data Store Write1/3
  0_boolean/1 -> Data Store Write/3, Data Store Write/2
  1_boolean/1 -> Data Store Write/1
  Data Store Read4/1 -> Sum/1
  Data Store Read1/1 -> Sum/2
  Sum/1 -> Discrete PI Controller with anti-windup & reset/1
  Data Store Read2/1 -> Discrete PI Controller with anti-windup & reset/2
  Data Store Read2/2 -> Product/1
  Data Store Read2/3 -> Product/2
  Product/1 -> Discrete PI Controller with anti-windup & reset/3
  Discrete PI Controller with anti-windup & reset/1 -> Truth Table/2(DutyReq)
  Truth Table/4(SWOCTRLcode) -> Data Store Write1/4
  Truth Table/5(OUTMASKcode) -> Data Store Write1/5
  Constant/1 -> Discrete PI Controller with anti-windup & reset/4, Discrete PI Controller with anti-windup & reset/5

== system BLDC_Ctrl_MBD/State Machine Task/State Functions/ReadyFunc ==
  ReadyFunc : TriggerPort  TriggerType=function-call  VariantControl=Variant
  Data Store Write : DataStoreWrite  DataStoreName=varPeripherals  DataStoreElements=varPeripherals.varLED.LEDR#varPeripherals.varLED.LEDG#varPeripherals.varLED.LEDB
  Data Store Write1 : DataStoreWrite  DataStoreName=varBLDC  DataStoreElements=varBLDC.varDuty.DutyA#varBLDC.varDuty.DutyB#varBLDC.varDuty.DutyC#varBLDC.varHallCalc.HallStart#varBLDC.varHallCalc.HallEnd
  boolean : Constant  Value=0  OutDataTypeStr=boolean
  boolean1 : Constant  OutDataTypeStr=boolean
  single : Constant  Value=0  OutDataTypeStr=single
  uint32 : Constant  Value=0  OutDataTypeStr=uint32
  wires:
  boolean1/1 -> Data Store Write/3, Data Store Write/1
  boolean/1 -> Data Store Write/2
  single/1 -> Data Store Write1/1, Data Store Write1/3, Data Store Write1/2
  uint32/1 -> Data Store Write1/5, Data Store Write1/4

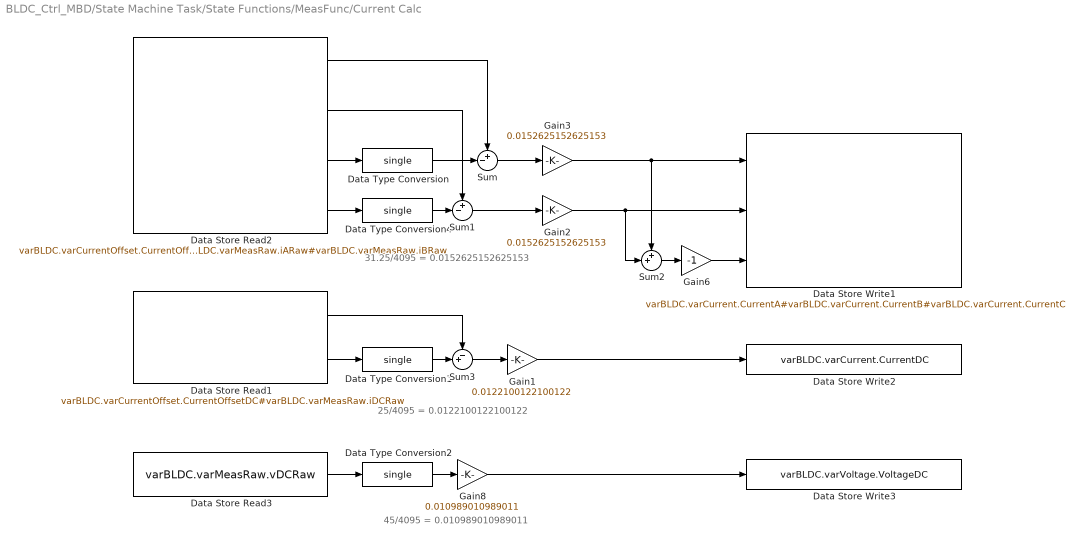
== system BLDC_Ctrl_MBD/State Machine Task/State Functions/MeasFunc/Current Calc ==
  note: 25/4095 = 0.0122100122100122
  note: 45/4095 = 0.010989010989011
  note: 31.25/4095 = 0.0152625152625153
  Data Store Read1 : DataStoreRead  DataStoreName=varBLDC  DataStoreElements=varBLDC.varCurrentOffset.CurrentOffsetDC#varBLDC.varMeasRaw.iDCRaw
  Data Store Read2 : DataStoreRead  DataStoreName=varBLDC  DataStoreElements=varBLDC.varCurrentOffset.CurrentOffsetA#varBLDC.varCurrentOffset.CurrentOffsetB#varBLDC.varMeasRaw.iARaw#varBLDC.varMeasRaw.iBRaw
  Data Store Read3 : DataStoreRead  DataStoreName=varBLDC  DataStoreElements=varBLDC.varMeasRaw.vDCRaw
  Data Store Write1 : DataStoreWrite  DataStoreName=varBLDC  DataStoreElements=varBLDC.varCurrent.CurrentA#varBLDC.varCurrent.CurrentB#varBLDC.varCurrent.CurrentC
  Data Store Write2 : DataStoreWrite  DataStoreName=varBLDC  DataStoreElements=varBLDC.varCurrent.CurrentDC
  Data Store Write3 : DataStoreWrite  DataStoreName=varBLDC  DataStoreElements=varBLDC.varVoltage.VoltageDC
  Data Type Conversion{,1..2,4} (4 alike) : DataTypeConversion  OutDataTypeStr=single
  Gain1 : Gain  Gain=0.0122100122100122  OutDataTypeStr=single
  Gain2 : Gain  Gain=0.0152625152625153  OutDataTypeStr=single
  Gain3 : Gain  Gain=0.0152625152625153  OutDataTypeStr=single
  Gain6 : Gain  Gain=-1  OutDataTypeStr=single
  Gain8 : Gain  Gain=0.010989010989011  OutDataTypeStr=single
  Sum : Sum  Inputs=+-|
  Sum1 : Sum  Inputs=+-|
  Sum2 : Sum  Inputs=++|
  Sum3 : Sum  Inputs=-+|
  wires:
  Data Store Read2/1 -> Sum/1
  Data Store Read2/3 -> Data Type Conversion/1
  Data Type Conversion2/1 -> Gain8/1
  Data Store Read1/1 -> Sum3/1
  Gain3/1 -> Data Store Write1/1, Sum2/1
  Gain1/1 -> Data Store Write2/1
  Sum1/1 -> Gain2/1
  Gain8/1 -> Data Store Write3/1
  Sum3/1 -> Gain1/1
  Data Store Read1/2 -> Data Type Conversion1/1
  Data Type Conversion1/1 -> Sum3/2
  Gain6/1 -> Data Store Write1/3
  Data Type Conversion4/1 -> Sum1/2
  Data Store Read2/4 -> Data Type Conversion4/1
  Sum/1 -> Gain3/1
  Sum2/1 -> Gain6/1
  Data Type Conversion/1 -> Sum/2
  Data Store Read3/1 -> Data Type Conversion2/1
  Gain2/1 -> Sum2/2, Data Store Write1/2
  Data Store Read2/2 -> Sum1/1

== system BLDC_Ctrl_MBD/State Machine Task/State Functions/MeasFunc/Hall Calc ==
  Data Store Read : DataStoreRead  DataStoreName=varBLDC  DataStoreElements=varBLDC.varHall.HallA#varBLDC.varHall.HallB#varBLDC.varHall.HallC
  Data Store Write5 : DataStoreWrite  DataStoreName=varBLDC  DataStoreElements=varBLDC.varHallCalc.HallXOR#varBLDC.varHallCalc.HallEdgeEvent#varBLDC.varHallCalc.HallSum
  Subsystem : Subsystem
  wires:
  Data Store Read/1 -> Subsystem/1(In1)
  Data Store Read/2 -> Subsystem/2(In2)
  Data Store Read/3 -> Subsystem/3(In3)
  Subsystem/1(Out1) -> Data Store Write5/1
  Subsystem/2(Out2) -> Data Store Write5/2
  Subsystem/3(Out3) -> Data Store Write5/3

== system BLDC_Ctrl_MBD/State Machine Task/State Functions/MeasFunc/Speed Calc ==
  Data Store Read1 : DataStoreRead  DataStoreName=varBLDC  DataStoreElements=varBLDC.varHallCalc.HallEnd
  Data Store Read2 : DataStoreRead  DataStoreName=varBLDC  DataStoreElements=varBLDC.varHallCalc.HallStart
  If : If  NumInputs=2  IfExpression=u1 < u2  ElseIfExpressions=u1 == u2
  If Action Subsystem : Subsystem  TreatAsAtomicUnit=on
  If Action Subsystem1 : Subsystem  TreatAsAtomicUnit=on
  If Action Subsystem2 : Subsystem  TreatAsAtomicUnit=on
  wires:
  If/3 -> If Action Subsystem1/Action
  Data Store Read2/1 -> If/1
  Data Store Read1/1 -> If/2
  If/1 -> If Action Subsystem/Action
  If/2 -> If Action Subsystem2/Action

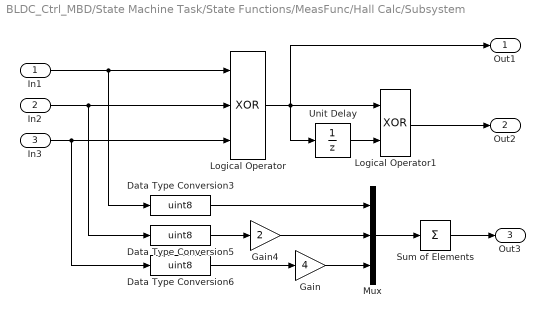
== system BLDC_Ctrl_MBD/State Machine Task/State Functions/MeasFunc/Hall Calc/Subsystem ==
  In1 : Inport
  In2 : Inport  Port=2
  In3 : Inport  Port=3
  Data Type Conversion3 : DataTypeConversion  OutDataTypeStr=uint8
  Data Type Conversion5 : DataTypeConversion  OutDataTypeStr=uint8
  Data Type Conversion6 : DataTypeConversion  OutDataTypeStr=uint8
  Gain : Gain  Gain=4  OutDataTypeStr=uint8
  Gain4 : Gain  Gain=2  OutDataTypeStr=uint8
  Logical Operator : Logic  Operator=XOR  Inputs=3  AllPortsSameDT=off  OutDataTypeStr=boolean
  Logical Operator1 : Logic  Operator=XOR  AllPortsSameDT=off  OutDataTypeStr=boolean
  Mux : Mux  Inputs=3
  Sum of Elements : Sum  Inputs=+
  Unit Delay : UnitDelay  SampleTime=-1  HasFrameUpgradeWarning=on
  Out1 : Outport
  Out2 : Outport  Port=2
  Out3 : Outport  Port=3
  wires:
  Gain4/1 -> Mux/2
  Unit Delay/1 -> Logical Operator1/2
  Logical Operator/1 -> Out1/1, Unit Delay/1, Logical Operator1/1
  In3/1 -> Data Type Conversion6/1, Logical Operator/3
  Data Type Conversion6/1 -> Gain/1
  Data Type Conversion3/1 -> Mux/1
  Gain/1 -> Mux/3
  In1/1 -> Data Type Conversion3/1, Logical Operator/1
  Mux/1 -> Sum of Elements/1
  Data Type Conversion5/1 -> Gain4/1
  In2/1 -> Data Type Conversion5/1, Logical Operator/2
  Sum of Elements/1 -> Out3/1
  Logical Operator1/1 -> Out2/1

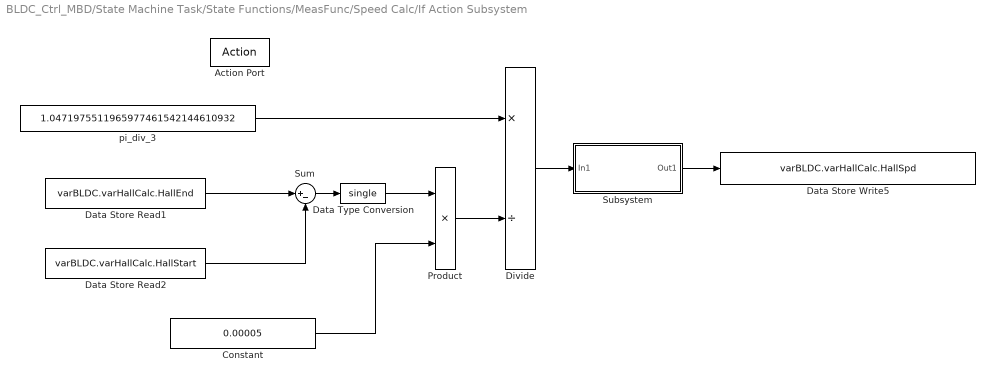
== system BLDC_Ctrl_MBD/State Machine Task/State Functions/MeasFunc/Speed Calc/If Action Subsystem ==
  Action Port : ActionPort  ActionPortLabel=if(u1 < u2)
  Constant : Constant  Value=0.00005  OutDataTypeStr=single
  Data Store Read1 : DataStoreRead  DataStoreName=varBLDC  DataStoreElements=varBLDC.varHallCalc.HallEnd
  Data Store Read2 : DataStoreRead  DataStoreName=varBLDC  DataStoreElements=varBLDC.varHallCalc.HallStart
  Data Store Write5 : DataStoreWrite  DataStoreName=varBLDC  DataStoreElements=varBLDC.varHallCalc.HallSpd
  Data Type Conversion : DataTypeConversion  OutDataTypeStr=single
  Divide : Product  Inputs=*/
  Product : Product
  Subsystem : Subsystem
  Sum : Sum  Inputs=|+-
  pi_div_3 : Constant  Value=1.0471975511965977461542144610932  OutDataTypeStr=single
  wires:
  Data Store Read1/1 -> Sum/1
  Data Store Read2/1 -> Sum/2
  pi_div_3/1 -> Divide/1
  Sum/1 -> Data Type Conversion/1
  Data Type Conversion/1 -> Product/1
  Divide/1 -> Subsystem/1(In1)
  Product/1 -> Divide/2
  Constant/1 -> Product/2
  Subsystem/1(Out1) -> Data Store Write5/1

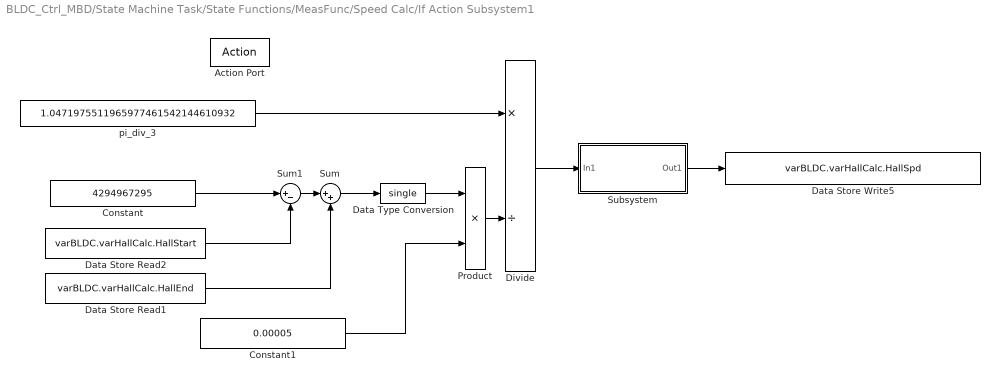
== system BLDC_Ctrl_MBD/State Machine Task/State Functions/MeasFunc/Speed Calc/If Action Subsystem1 ==
  Action Port : ActionPort  ActionPortLabel=else
  Constant : Constant  Value=4294967295  OutDataTypeStr=uint32
  Constant1 : Constant  Value=0.00005  OutDataTypeStr=single
  Data Store Read1 : DataStoreRead  DataStoreName=varBLDC  DataStoreElements=varBLDC.varHallCalc.HallEnd
  Data Store Read2 : DataStoreRead  DataStoreName=varBLDC  DataStoreElements=varBLDC.varHallCalc.HallStart
  Data Store Write5 : DataStoreWrite  DataStoreName=varBLDC  DataStoreElements=varBLDC.varHallCalc.HallSpd
  Data Type Conversion : DataTypeConversion  OutDataTypeStr=single
  Divide : Product  Inputs=*/
  Product : Product
  Subsystem : Subsystem
  Sum : Sum  Inputs=|++
  Sum1 : Sum  Inputs=|+-
  pi_div_3 : Constant  Value=1.0471975511965977461542144610932  OutDataTypeStr=single
  wires:
  Data Type Conversion/1 -> Product/1
  Data Store Read1/1 -> Sum/2
  pi_div_3/1 -> Divide/1
  Constant/1 -> Sum1/1
  Data Store Read2/1 -> Sum1/2
  Sum1/1 -> Sum/1
  Sum/1 -> Data Type Conversion/1
  Constant1/1 -> Product/2
  Product/1 -> Divide/2
  Divide/1 -> Subsystem/1(In1)
  Subsystem/1(Out1) -> Data Store Write5/1

== system BLDC_Ctrl_MBD/State Machine Task/State Functions/MeasFunc/Speed Calc/If Action Subsystem2 ==
  Action Port : ActionPort  ActionPortLabel=elseif(u1 == u2)
  Constant : Constant  Value=0  OutDataTypeStr=single
  Data Store Write5 : DataStoreWrite  DataStoreName=varBLDC  DataStoreElements=varBLDC.varHallCalc.HallSpd
  wires:
  Constant/1 -> Data Store Write5/1

== system BLDC_Ctrl_MBD/State Machine Task/State Functions/MeasFunc/Speed Calc/If Action Subsystem/Subsystem ==
  In1 : Inport
  Constant1 : Constant  OutDataTypeStr=single
  Constant2 : Constant  Value=0.0001  OutDataTypeStr=single
  Data Store Read3 : DataStoreRead  DataStoreName=varBLDC  DataStoreElements=varBLDC.varHallCalc.HallSpd
  Product1 : Product
  Product2 : Product
  Sum1 : Sum  Inputs=|+-
  Sum2 : Sum  Inputs=|++
  Out1 : Outport
  wires:
  Sum1/1 -> Product1/2
  Constant2/1 -> Product2/1, Sum1/2
  Constant1/1 -> Sum1/1
  Product1/1 -> Sum2/1
  Data Store Read3/1 -> Product1/1
  Sum2/1 -> Out1/1
  Product2/1 -> Sum2/2
  In1/1 -> Product2/2

== system BLDC_Ctrl_MBD/State Machine Task/State Functions/MeasFunc/Speed Calc/If Action Subsystem1/Subsystem ==
  In1 : Inport
  Constant1 : Constant  OutDataTypeStr=single
  Constant2 : Constant  Value=0.0001  OutDataTypeStr=single
  Data Store Read3 : DataStoreRead  DataStoreName=varBLDC  DataStoreElements=varBLDC.varHallCalc.HallSpd
  Product1 : Product
  Product2 : Product
  Sum1 : Sum  Inputs=|+-
  Sum2 : Sum  Inputs=|++
  Out1 : Outport
  wires:
  Sum1/1 -> Product1/2
  Constant2/1 -> Product2/1, Sum1/2
  Constant1/1 -> Sum1/1
  Product1/1 -> Sum2/1
  Data Store Read3/1 -> Product1/1
  Sum2/1 -> Out1/1
  Product2/1 -> Sum2/2
  In1/1 -> Product2/2
